simulink model "Controller_HIL"  (R2024a)
settings: Solver=FixedStepDiscrete  StartTime=0.0  StopTime=inf  FixedStep=ts_controller  RelTol=1e-3
InitFcn:
  | mbd_s32k_consistency_checks(bdroot(gcs));
undefined symbols (not defined in the file): Battery, BMS_Controller_State, Charging_State, currentFactor, CV_Gain, DiscIntNeverNeededParam, I_cc, LQFP, MaxCellVoltThrsld, noCurrent, Ns_Module, NumModules, OverCellVoltageLimit, SOCInit, SRE, ts_controller, ts_system, UnderCellVoltageLimit, voltThreshold
libraries: mbd_s32k1xx_ec_toolbox x104, etargetslib x95, mbd_bcc_ec_toolbox x30, hdlsllib x11, simulink x6, sharedTrackingLibrary x2
(part 2 of 4)

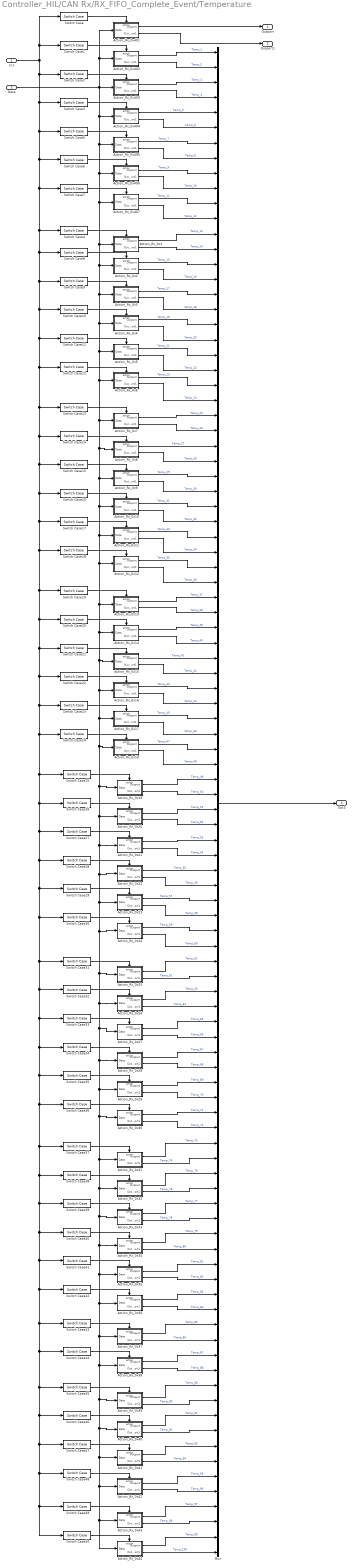
== system Controller_HIL/CAN Rx/RX_FIFO_Complete_Event/Temperature ==
  In1 : Inport
  Data : Inport  Port=2
  Action_Rx_0x1 : Subsystem  TreatAsAtomicUnit=on
  Action_Rx_0x10 : Subsystem  TreatAsAtomicUnit=on
  Action_Rx_0x11 : Subsystem  TreatAsAtomicUnit=on
  Action_Rx_0x12 : Subsystem  TreatAsAtomicUnit=on
  Action_Rx_0x13 : Subsystem  TreatAsAtomicUnit=on
  Action_Rx_0x14 : Subsystem  TreatAsAtomicUnit=on
  Action_Rx_0x15 : Subsystem  TreatAsAtomicUnit=on
  Action_Rx_0x16 : Subsystem  TreatAsAtomicUnit=on
  Action_Rx_0x17 : Subsystem  TreatAsAtomicUnit=on
  Action_Rx_0x18 : Subsystem  TreatAsAtomicUnit=on
  Action_Rx_0x19 : Subsystem  TreatAsAtomicUnit=on
  Action_Rx_0x2 : Subsystem  TreatAsAtomicUnit=on
  Action_Rx_0x20 : Subsystem  TreatAsAtomicUnit=on
  Action_Rx_0x21 : Subsystem  TreatAsAtomicUnit=on
  Action_Rx_0x22 : Subsystem  TreatAsAtomicUnit=on
  Action_Rx_0x23 : Subsystem  TreatAsAtomicUnit=on
  Action_Rx_0x24 : Subsystem  TreatAsAtomicUnit=on
  Action_Rx_0x25 : Subsystem  TreatAsAtomicUnit=on
  Action_Rx_0x26 : Subsystem  TreatAsAtomicUnit=on
  Action_Rx_0x27 : Subsystem  TreatAsAtomicUnit=on
  Action_Rx_0x28 : Subsystem  TreatAsAtomicUnit=on
  Action_Rx_0x29 : Subsystem  TreatAsAtomicUnit=on
  Action_Rx_0x3 : Subsystem  TreatAsAtomicUnit=on
  Action_Rx_0x30 : Subsystem  TreatAsAtomicUnit=on
  Action_Rx_0x31 : Subsystem  TreatAsAtomicUnit=on
  Action_Rx_0x32 : Subsystem  TreatAsAtomicUnit=on
  Action_Rx_0x33 : Subsystem  TreatAsAtomicUnit=on
  Action_Rx_0x34 : Subsystem  TreatAsAtomicUnit=on
  Action_Rx_0x35 : Subsystem  TreatAsAtomicUnit=on
  Action_Rx_0x36 : Subsystem  TreatAsAtomicUnit=on
  Action_Rx_0x37 : Subsystem  TreatAsAtomicUnit=on
  Action_Rx_0x38 : Subsystem  TreatAsAtomicUnit=on
  Action_Rx_0x39 : Subsystem  TreatAsAtomicUnit=on
  Action_Rx_0x4 : Subsystem  TreatAsAtomicUnit=on
  Action_Rx_0x40 : Subsystem  TreatAsAtomicUnit=on
  Action_Rx_0x401 : Subsystem  TreatAsAtomicUnit=on
  Action_Rx_0x402 : Subsystem  TreatAsAtomicUnit=on
  Action_Rx_0x403 : Subsystem  TreatAsAtomicUnit=on
  Action_Rx_0x404 : Subsystem  TreatAsAtomicUnit=on
  Action_Rx_0x405 : Subsystem  TreatAsAtomicUnit=on
  Action_Rx_0x406 : Subsystem  TreatAsAtomicUnit=on
  Action_Rx_0x407 : Subsystem  TreatAsAtomicUnit=on
  Action_Rx_0x41 : Subsystem  TreatAsAtomicUnit=on
  Action_Rx_0x42 : Subsystem  TreatAsAtomicUnit=on
  Action_Rx_0x43 : Subsystem  TreatAsAtomicUnit=on
  Action_Rx_0x44 : Subsystem  TreatAsAtomicUnit=on
  Action_Rx_0x5 : Subsystem  TreatAsAtomicUnit=on
  Action_Rx_0x6 : Subsystem  TreatAsAtomicUnit=on
  Action_Rx_0x7 : Subsystem  TreatAsAtomicUnit=on
  Action_Rx_0x8 : Subsystem  TreatAsAtomicUnit=on
  Action_Rx_0x9 : Subsystem  TreatAsAtomicUnit=on
  Mux : Mux  Inputs=100
  Switch Case : SwitchCase  CaseConditions={hex2dec('401')}  ShowDefaultCase=off
  Switch Case1 : SwitchCase  CaseConditions={hex2dec('402')}  ShowDefaultCase=off
  Switch Case10 : SwitchCase  CaseConditions={hex2dec('411')}  ShowDefaultCase=off
  Switch Case11 : SwitchCase  CaseConditions={hex2dec('412')}  ShowDefaultCase=off
  Switch Case12 : SwitchCase  CaseConditions={hex2dec('413')}  ShowDefaultCase=off
  Switch Case13 : SwitchCase  CaseConditions={hex2dec('414')}  ShowDefaultCase=off
  Switch Case14 : SwitchCase  CaseConditions={hex2dec('415')}  ShowDefaultCase=off
  Switch Case15 : SwitchCase  CaseConditions={hex2dec('416')}  ShowDefaultCase=off
  Switch Case16 : SwitchCase  CaseConditions={hex2dec('417')}  ShowDefaultCase=off
  Switch Case17 : SwitchCase  CaseConditions={hex2dec('418')}  ShowDefaultCase=off
  Switch Case18 : SwitchCase  CaseConditions={hex2dec('419')}  ShowDefaultCase=off
  Switch Case19 : SwitchCase  CaseConditions={hex2dec('420')}  ShowDefaultCase=off
  Switch Case2 : SwitchCase  CaseConditions={hex2dec('403')}  ShowDefaultCase=off
  Switch Case20 : SwitchCase  CaseConditions={hex2dec('421')}  ShowDefaultCase=off
  Switch Case21 : SwitchCase  CaseConditions={hex2dec('422')}  ShowDefaultCase=off
  Switch Case22 : SwitchCase  CaseConditions={hex2dec('423')}  ShowDefaultCase=off
  Switch Case23 : SwitchCase  CaseConditions={hex2dec('424')}  ShowDefaultCase=off
  Switch Case24 : SwitchCase  CaseConditions={hex2dec('425')}  ShowDefaultCase=off
  Switch Case25 : SwitchCase  CaseConditions={hex2dec('426')}  ShowDefaultCase=off
  Switch Case26 : SwitchCase  CaseConditions={hex2dec('427')}  ShowDefaultCase=off
  Switch Case27 : SwitchCase  CaseConditions={hex2dec('428')}  ShowDefaultCase=off
  Switch Case28 : SwitchCase  CaseConditions={hex2dec('429')}  ShowDefaultCase=off
  Switch Case29 : SwitchCase  CaseConditions={hex2dec('430')}  ShowDefaultCase=off
  Switch Case3 : SwitchCase  CaseConditions={hex2dec('404')}  ShowDefaultCase=off
  Switch Case30 : SwitchCase  CaseConditions={hex2dec('431')}  ShowDefaultCase=off
  Switch Case31 : SwitchCase  CaseConditions={hex2dec('432')}  ShowDefaultCase=off
  Switch Case32 : SwitchCase  CaseConditions={hex2dec('433')}  ShowDefaultCase=off
  Switch Case33 : SwitchCase  CaseConditions={hex2dec('434')}  ShowDefaultCase=off
  Switch Case34 : SwitchCase  CaseConditions={hex2dec('435')}  ShowDefaultCase=off
  Switch Case35 : SwitchCase  CaseConditions={hex2dec('436')}  ShowDefaultCase=off
  Switch Case36 : SwitchCase  CaseConditions={hex2dec('437')}  ShowDefaultCase=off
  Switch Case37 : SwitchCase  CaseConditions={hex2dec('438')}  ShowDefaultCase=off
  Switch Case38 : SwitchCase  CaseConditions={hex2dec('439')}  ShowDefaultCase=off
  Switch Case39 : SwitchCase  CaseConditions={hex2dec('440')}  ShowDefaultCase=off
  Switch Case4 : SwitchCase  CaseConditions={hex2dec('408')}  ShowDefaultCase=off
  Switch Case40 : SwitchCase  CaseConditions={hex2dec('441')}  ShowDefaultCase=off
  Switch Case41 : SwitchCase  CaseConditions={hex2dec('442')}  ShowDefaultCase=off
  Switch Case42 : SwitchCase  CaseConditions={hex2dec('443')}  ShowDefaultCase=off
  Switch Case43 : SwitchCase  CaseConditions={hex2dec('444')}  ShowDefaultCase=off
  Switch Case44 : SwitchCase  CaseConditions={hex2dec('445')}  ShowDefaultCase=off
  Switch Case45 : SwitchCase  CaseConditions={hex2dec('446')}  ShowDefaultCase=off
  Switch Case46 : SwitchCase  CaseConditions={hex2dec('447')}  ShowDefaultCase=off
  Switch Case47 : SwitchCase  CaseConditions={hex2dec('448')}  ShowDefaultCase=off
  Switch Case48 : SwitchCase  CaseConditions={hex2dec('449')}  ShowDefaultCase=off
  Switch Case49 : SwitchCase  CaseConditions={hex2dec('450')}  ShowDefaultCase=off
  Switch Case5 : SwitchCase  CaseConditions={hex2dec('405')}  ShowDefaultCase=off
  Switch Case50 : SwitchCase  CaseConditions={hex2dec('451')}  ShowDefaultCase=off
  Switch Case6 : SwitchCase  CaseConditions={hex2dec('406')}  ShowDefaultCase=off
  Switch Case7 : SwitchCase  CaseConditions={hex2dec('407')}  ShowDefaultCase=off
  Switch Case8 : SwitchCase  CaseConditions={hex2dec('409')}  ShowDefaultCase=off
  Switch Case9 : SwitchCase  CaseConditions={hex2dec('410')}  ShowDefaultCase=off
  Outport : Outport
  Outport1 : Outport  Port=2
  Out3 : Outport  Port=3
  wires:
  Action_Rx_0x35/1(Outport) -> Mux/81  "Temp_81"
  Action_Rx_0x19/2(Outport1) -> Mux/50  "Temp_50"
  Switch Case38/1 -> Action_Rx_0x32/Action
  In1/1 -> Switch Case3/1, Switch Case5/1, Switch Case6/1, Switch Case8/1, Switch Case9/1, Switch Case10/1, Switch Case11/1, Switch Case12/1, Switch Case13/1, Switch Case14/1, Switch Case15/1, Switch Case16/1, Switch Case18/1, Switch Case20/1, Switch Case21/1, Switch Case22/1, Switch Case23/1, Switch Case24/1, Switch Case25/1, Switch Case26/1, Switch Case28/1, Switch Case29/1, Switch Case31/1, Switch Case32/1, Switch Case33/1, Switch Case34/1, Switch Case35/1, Switch Case37/1, Switch Case38/1, Switch Case39/1, Switch Case40/1, Switch Case41/1, Switch Case45/1, Switch Case46/1, Switch Case48/1, Switch Case49/1, Switch Case50/1, Switch Case47/1, Switch Case44/1, Switch Case43/1, Switch Case42/1, Switch Case36/1, Switch Case30/1, Switch Case27/1, Switch Case19/1, Switch Case17/1, Switch Case4/1, Switch Case7/1, Switch Case2/1, Switch Case1/1, Switch Case/1
  Switch Case1/1 -> Action_Rx_0x402/Action
  Switch Case6/1 -> Action_Rx_0x406/Action
  Action_Rx_0x14/1(Outport) -> Mux/39  "Temp_39"
  Data/1 -> Action_Rx_0x405/1(Data), Action_Rx_0x406/1(Data), Action_Rx_0x3/1(Data), Action_Rx_0x4/1(Data), Action_Rx_0x5/1(Data), Action_Rx_0x7/1(Data), Action_Rx_0x8/1(Data), Action_Rx_0x9/1(Data), Action_Rx_0x10/1(Data), Action_Rx_0x11/1(Data), Action_Rx_0x12/1(Data), Action_Rx_0x13/1(Data), Action_Rx_0x14/1(Data), Action_Rx_0x15/1(Data), Action_Rx_0x16/1(Data), Action_Rx_0x17/1(Data), Action_Rx_0x18/1(Data), Action_Rx_0x19/1(Data), Action_Rx_0x20/1(Data), Action_Rx_0x21/1(Data), Action_Rx_0x22/1(Data), Action_Rx_0x23/1(Data), Action_Rx_0x24/1(Data), Action_Rx_0x25/1(Data), Action_Rx_0x26/1(Data), Action_Rx_0x27/1(Data), Action_Rx_0x28/1(Data), Action_Rx_0x29/1(Data), Action_Rx_0x30/1(Data), Action_Rx_0x31/1(Data), Action_Rx_0x32/1(Data), Action_Rx_0x33/1(Data), Action_Rx_0x34/1(Data), Action_Rx_0x35/1(Data), Action_Rx_0x36/1(Data), Action_Rx_0x37/1(Data), Action_Rx_0x39/1(Data), Action_Rx_0x40/1(Data), Action_Rx_0x41/1(Data), Action_Rx_0x42/1(Data), Action_Rx_0x43/1(Data), Action_Rx_0x44/1(Data), Action_Rx_0x38/1(Data), Action_Rx_0x6/1(Data), Action_Rx_0x2/1(Data), Action_Rx_0x1/1(Data), Action_Rx_0x407/1(Data), Action_Rx_0x404/1(Data), Action_Rx_0x403/1(Data), Action_Rx_0x402/1(Data), Action_Rx_0x401/1(Data)
  Switch Case43/1 -> Action_Rx_0x37/Action
  Action_Rx_0x13/1(Outport) -> Mux/37  "Temp_37"
  Switch Case2/1 -> Action_Rx_0x403/Action
  Action_Rx_0x34/1(Outport) -> Mux/79  "Temp_79"
  Action_Rx_0x5/1(Outport) -> Mux/21  "Temp_21"
  Action_Rx_0x44/2(Outport1) -> Mux/100  "Temp_100"
  Action_Rx_0x15/1(Outport) -> Mux/41  "Temp_41"
  Switch Case18/1 -> Action_Rx_0x12/Action
  Action_Rx_0x31/1(Outport) -> Mux/73  "Temp_73"
  Switch Case7/1 -> Action_Rx_0x407/Action
  Switch Case47/1 -> Action_Rx_0x41/Action
  Switch Case14/1 -> Action_Rx_0x8/Action
  Action_Rx_0x405/1(Outport) -> Mux/7  "Temp_7"
  Switch Case20/1 -> Action_Rx_0x14/Action
  Action_Rx_0x4/1(Outport) -> Mux/19  "Temp_19"
  Action_Rx_0x402/2(Outport1) -> Mux/2  "Temp_2"
  Switch Case3/1 -> Action_Rx_0x404/Action
  Action_Rx_0x20/1(Outport) -> Mux/51  "Temp_51"
  Action_Rx_0x17/2(Outport1) -> Mux/46  "Temp_46"
  Switch Case8/1 -> Action_Rx_0x2/Action
  Action_Rx_0x21/1(Outport) -> Mux/53  "Temp_53"
  Switch Case50/1 -> Action_Rx_0x44/Action
  Action_Rx_0x43/2(Outport1) -> Mux/98  "Temp_98"
  Mux/1 -> Out3/1
  Action_Rx_0x40/2(Outport1) -> Mux/92  "Temp_92"
  Switch Case13/1 -> Action_Rx_0x7/Action
  Action_Rx_0x32/1(Outport) -> Mux/75  "Temp_75"
  Switch Case21/1 -> Action_Rx_0x15/Action
  Switch Case35/1 -> Action_Rx_0x29/Action
  Action_Rx_0x406/2(Outport1) -> Mux/10  "Temp_10"
  Action_Rx_0x25/1(Outport) -> Mux/61  "Temp_61"
  Switch Case32/1 -> Action_Rx_0x26/Action
  Action_Rx_0x403/1(Outport) -> Mux/3  "Temp_3"
  Action_Rx_0x6/1(Outport) -> Mux/23  "Temp_23"
  Action_Rx_0x36/2(Outport1) -> Mux/84  "Temp_84"
  Action_Rx_0x1/2(Outport1) -> Mux/14  "Temp_14"
  Action_Rx_0x18/2(Outport1) -> Mux/48  "Temp_48"
  Action_Rx_0x404/2(Outport1) -> Mux/6  "Temp_6"
  Action_Rx_0x2/2(Outport1) -> Mux/16  "Temp_16"
  Action_Rx_0x405/2(Outport1) -> Mux/8  "Temp_8"
  Action_Rx_0x42/2(Outport1) -> Mux/96  "Temp_96"
  Action_Rx_0x9/2(Outport1) -> Mux/30  "Temp_30"
  Action_Rx_0x13/2(Outport1) -> Mux/38  "Temp_38"
  Action_Rx_0x15/2(Outport1) -> Mux/42  "Temp_42"
  Switch Case16/1 -> Action_Rx_0x10/Action
  Action_Rx_0x34/2(Outport1) -> Mux/80  "Temp_80"
  Switch Case9/1 -> Action_Rx_0x3/Action
  Switch Case27/1 -> Action_Rx_0x21/Action
  Switch Case30/1 -> Action_Rx_0x24/Action
  Action_Rx_0x4/2(Outport1) -> Mux/20  "Temp_20"
  Action_Rx_0x16/2(Outport1) -> Mux/44  "Temp_44"
  Switch Case31/1 -> Action_Rx_0x25/Action
  Action_Rx_0x407/1(Outport) -> Mux/11  "Temp_11"
  Switch Case45/1 -> Action_Rx_0x39/Action
  Switch Case33/1 -> Action_Rx_0x27/Action
  Action_Rx_0x38/1(Outport) -> Mux/87  "Temp_87"
  Switch Case22/1 -> Action_Rx_0x16/Action
  Switch Case12/1 -> Action_Rx_0x6/Action
  Switch Case41/1 -> Action_Rx_0x35/Action
  Switch Case19/1 -> Action_Rx_0x13/Action
  Action_Rx_0x403/2(Outport1) -> Mux/4  "Temp_4"
  Switch Case29/1 -> Action_Rx_0x23/Action
  Action_Rx_0x22/1(Outport) -> Mux/55  "Temp_55"
  Switch Case39/1 -> Action_Rx_0x33/Action
  Action_Rx_0x407/2(Outport1) -> Mux/12  "Temp_12"
  Switch Case/1 -> Action_Rx_0x401/Action
  Action_Rx_0x20/2(Outport1) -> Mux/52  "Temp_52"
  Action_Rx_0x16/1(Outport) -> Mux/43  "Temp_43"
  Action_Rx_0x10/1(Outport) -> Mux/31  "Temp_31"
  Switch Case4/1 -> Action_Rx_0x1/Action
  Action_Rx_0x28/1(Outport) -> Mux/67  "Temp_67"
  Switch Case17/1 -> Action_Rx_0x11/Action
  Switch Case46/1 -> Action_Rx_0x40/Action
  Action_Rx_0x22/2(Outport1) -> Mux/56  "Temp_56"
  Action_Rx_0x26/1(Outport) -> Mux/63  "Temp_63"
  Action_Rx_0x7/2(Outport1) -> Mux/26  "Temp_26"
  Action_Rx_0x26/2(Outport1) -> Mux/64  "Temp_64"
  Action_Rx_0x3/2(Outport1) -> Mux/18  "Temp_18"
  Action_Rx_0x38/2(Outport1) -> Mux/88  "Temp_88"
  Switch Case49/1 -> Action_Rx_0x43/Action
  Action_Rx_0x41/2(Outport1) -> Mux/94  "Temp_94"
  Action_Rx_0x23/1(Outport) -> Mux/57  "Temp_57"
  Action_Rx_0x25/2(Outport1) -> Mux/62  "Temp_62"
  Action_Rx_0x37/1(Outport) -> Mux/85  "Temp_85"
  Action_Rx_0x27/2(Outport1) -> Mux/66  "Temp_66"
  Action_Rx_0x35/2(Outport1) -> Mux/82  "Temp_82"
  Action_Rx_0x33/1(Outport) -> Mux/77  "Temp_77"
  Action_Rx_0x29/1(Outport) -> Mux/69  "Temp_69"
  Action_Rx_0x8/1(Outport) -> Mux/27  "Temp_27"
  Action_Rx_0x404/1(Outport) -> Mux/5  "Temp_5"
  Action_Rx_0x30/1(Outport) -> Mux/71  "Temp_71"
  Switch Case5/1 -> Action_Rx_0x405/Action
  Switch Case26/1 -> Action_Rx_0x20/Action
  Action_Rx_0x28/2(Outport1) -> Mux/68  "Temp_68"
  Switch Case48/1 -> Action_Rx_0x42/Action
  Action_Rx_0x39/2(Outport1) -> Mux/90  "Temp_90"
  Action_Rx_0x406/1(Outport) -> Mux/9  "Temp_9"
  Action_Rx_0x9/1(Outport) -> Mux/29  "Temp_29"
  Action_Rx_0x7/1(Outport) -> Mux/25  "Temp_25"
  Action_Rx_0x24/1(Outport) -> Mux/59  "Temp_59"
  Switch Case25/1 -> Action_Rx_0x19/Action
  Action_Rx_0x32/2(Outport1) -> Mux/76  "Temp_76"
  Action_Rx_0x1/1(Outport) -> Mux/13  "Temp_13"
  Action_Rx_0x29/2(Outport1) -> Mux/70  "Temp_70"
  Action_Rx_0x31/2(Outport1) -> Mux/74  "Temp_74"
  Switch Case42/1 -> Action_Rx_0x36/Action
  Switch Case23/1 -> Action_Rx_0x17/Action
  Action_Rx_0x33/2(Outport1) -> Mux/78  "Temp_78"
  Action_Rx_0x36/1(Outport) -> Mux/83  "Temp_83"
  Switch Case37/1 -> Action_Rx_0x31/Action
  Switch Case44/1 -> Action_Rx_0x38/Action
  Switch Case24/1 -> Action_Rx_0x18/Action
  Action_Rx_0x21/2(Outport1) -> Mux/54  "Temp_54"
  Action_Rx_0x11/1(Outport) -> Mux/33  "Temp_33"
  Action_Rx_0x401/2(Outport1) -> Outport1/1
  Action_Rx_0x41/1(Outport) -> Mux/93  "Temp_93"
  Switch Case34/1 -> Action_Rx_0x28/Action
  Switch Case36/1 -> Action_Rx_0x30/Action
  Action_Rx_0x37/2(Outport1) -> Mux/86  "Temp_86"
  Action_Rx_0x27/1(Outport) -> Mux/65  "Temp_65"
  Action_Rx_0x44/1(Outport) -> Mux/99  "Temp_99"
  Action_Rx_0x14/2(Outport1) -> Mux/40  "Temp_40"
  Action_Rx_0x40/1(Outport) -> Mux/91  "Temp_91"
  Action_Rx_0x402/1(Outport) -> Mux/1  "Temp_1"
  Switch Case15/1 -> Action_Rx_0x9/Action
  Action_Rx_0x12/1(Outport) -> Mux/35  "Temp_35"
  Switch Case28/1 -> Action_Rx_0x22/Action
  Switch Case40/1 -> Action_Rx_0x34/Action
  Action_Rx_0x24/2(Outport1) -> Mux/60  "Temp_60"
  Action_Rx_0x23/2(Outport1) -> Mux/58  "Temp_58"
  Action_Rx_0x17/1(Outport) -> Mux/45  "Temp_45"
  Action_Rx_0x18/1(Outport) -> Mux/47  "Temp_47"
  Action_Rx_0x8/2(Outport1) -> Mux/28  "Temp_28"
  Action_Rx_0x6/2(Outport1) -> Mux/24  "Temp_24"
  Action_Rx_0x39/1(Outport) -> Mux/89  "Temp_89"
  Action_Rx_0x5/2(Outport1) -> Mux/22  "Temp_22"
  Action_Rx_0x43/1(Outport) -> Mux/97  "Temp_97"
  Action_Rx_0x42/1(Outport) -> Mux/95  "Temp_95"
  Action_Rx_0x19/1(Outport) -> Mux/49  "Temp_49"
  Action_Rx_0x30/2(Outport1) -> Mux/72  "Temp_72"
  Switch Case11/1 -> Action_Rx_0x5/Action
  Action_Rx_0x2/1(Outport) -> Mux/15  "Temp_15"
  Action_Rx_0x3/1(Outport) -> Mux/17  "Temp_17"
  Action_Rx_0x11/2(Outport1) -> Mux/34  "Temp_34"
  Switch Case10/1 -> Action_Rx_0x4/Action
  Action_Rx_0x12/2(Outport1) -> Mux/36  "Temp_36"
  Action_Rx_0x10/2(Outport1) -> Mux/32  "Temp_32"
  Action_Rx_0x401/1(Outport) -> Outport/1

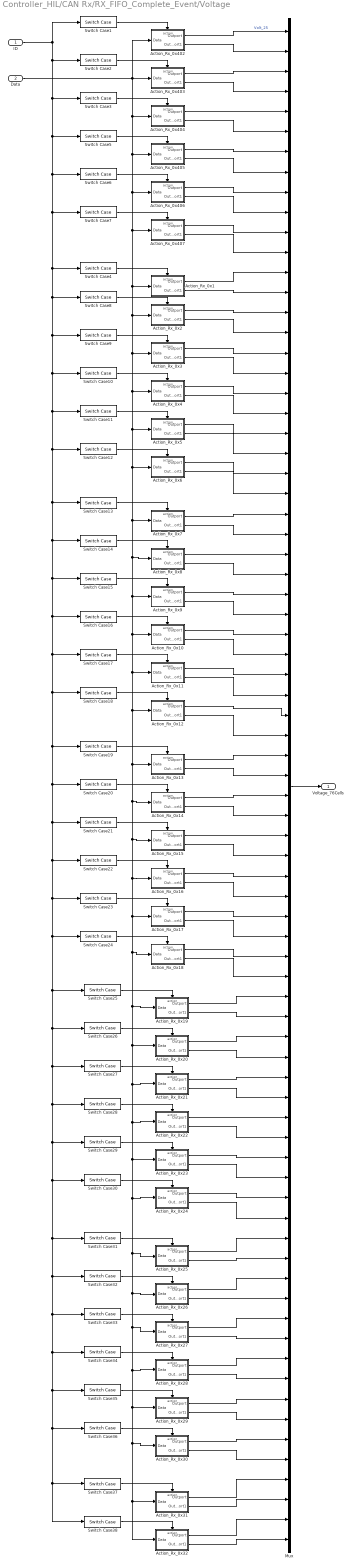
== system Controller_HIL/CAN Rx/RX_FIFO_Complete_Event/Voltage ==
  ID : Inport
  Data : Inport  Port=2
  Action_Rx_0x1 : Subsystem  TreatAsAtomicUnit=on
  Action_Rx_0x10 : Subsystem  TreatAsAtomicUnit=on
  Action_Rx_0x11 : Subsystem  TreatAsAtomicUnit=on
  Action_Rx_0x12 : Subsystem  TreatAsAtomicUnit=on
  Action_Rx_0x13 : Subsystem  TreatAsAtomicUnit=on
  Action_Rx_0x14 : Subsystem  TreatAsAtomicUnit=on
  Action_Rx_0x15 : Subsystem  TreatAsAtomicUnit=on
  Action_Rx_0x16 : Subsystem  TreatAsAtomicUnit=on
  Action_Rx_0x17 : Subsystem  TreatAsAtomicUnit=on
  Action_Rx_0x18 : Subsystem  TreatAsAtomicUnit=on
  Action_Rx_0x19 : Subsystem  TreatAsAtomicUnit=on
  Action_Rx_0x2 : Subsystem  TreatAsAtomicUnit=on
  Action_Rx_0x20 : Subsystem  TreatAsAtomicUnit=on
  Action_Rx_0x21 : Subsystem  TreatAsAtomicUnit=on
  Action_Rx_0x22 : Subsystem  TreatAsAtomicUnit=on
  Action_Rx_0x23 : Subsystem  TreatAsAtomicUnit=on
  Action_Rx_0x24 : Subsystem  TreatAsAtomicUnit=on
  Action_Rx_0x25 : Subsystem  TreatAsAtomicUnit=on
  Action_Rx_0x26 : Subsystem  TreatAsAtomicUnit=on
  Action_Rx_0x27 : Subsystem  TreatAsAtomicUnit=on
  Action_Rx_0x28 : Subsystem  TreatAsAtomicUnit=on
  Action_Rx_0x29 : Subsystem  TreatAsAtomicUnit=on
  Action_Rx_0x3 : Subsystem  TreatAsAtomicUnit=on
  Action_Rx_0x30 : Subsystem  TreatAsAtomicUnit=on
  Action_Rx_0x31 : Subsystem  TreatAsAtomicUnit=on
  Action_Rx_0x32 : Subsystem  TreatAsAtomicUnit=on
  Action_Rx_0x4 : Subsystem  TreatAsAtomicUnit=on
  Action_Rx_0x402 : Subsystem  TreatAsAtomicUnit=on
  Action_Rx_0x403 : Subsystem  TreatAsAtomicUnit=on
  Action_Rx_0x404 : Subsystem  TreatAsAtomicUnit=on
  Action_Rx_0x405 : Subsystem  TreatAsAtomicUnit=on
  Action_Rx_0x406 : Subsystem  TreatAsAtomicUnit=on
  Action_Rx_0x407 : Subsystem  TreatAsAtomicUnit=on
  Action_Rx_0x5 : Subsystem  TreatAsAtomicUnit=on
  Action_Rx_0x6 : Subsystem  TreatAsAtomicUnit=on
  Action_Rx_0x7 : Subsystem  TreatAsAtomicUnit=on
  Action_Rx_0x8 : Subsystem  TreatAsAtomicUnit=on
  Action_Rx_0x9 : Subsystem  TreatAsAtomicUnit=on
  Mux : Mux  Inputs=76
  Switch Case1 : SwitchCase  CaseConditions={hex2dec('452')}  ShowDefaultCase=off
  Switch Case10 : SwitchCase  CaseConditions={hex2dec('461')}  ShowDefaultCase=off
  Switch Case11 : SwitchCase  CaseConditions={hex2dec('462')}  ShowDefaultCase=off
  Switch Case12 : SwitchCase  CaseConditions={hex2dec('463')}  ShowDefaultCase=off
  Switch Case13 : SwitchCase  CaseConditions={hex2dec('464')}  ShowDefaultCase=off
  Switch Case14 : SwitchCase  CaseConditions={hex2dec('465')}  ShowDefaultCase=off
  Switch Case15 : SwitchCase  CaseConditions={hex2dec('466')}  ShowDefaultCase=off
  Switch Case16 : SwitchCase  CaseConditions={hex2dec('467')}  ShowDefaultCase=off
  Switch Case17 : SwitchCase  CaseConditions={hex2dec('468')}  ShowDefaultCase=off
  Switch Case18 : SwitchCase  CaseConditions={hex2dec('469')}  ShowDefaultCase=off
  Switch Case19 : SwitchCase  CaseConditions={hex2dec('470')}  ShowDefaultCase=off
  Switch Case2 : SwitchCase  CaseConditions={hex2dec('453')}  ShowDefaultCase=off
  Switch Case20 : SwitchCase  CaseConditions={hex2dec('471')}  ShowDefaultCase=off
  Switch Case21 : SwitchCase  CaseConditions={hex2dec('472')}  ShowDefaultCase=off
  Switch Case22 : SwitchCase  CaseConditions={hex2dec('473')}  ShowDefaultCase=off
  Switch Case23 : SwitchCase  CaseConditions={hex2dec('474')}  ShowDefaultCase=off
  Switch Case24 : SwitchCase  CaseConditions={hex2dec('475')}  ShowDefaultCase=off
  Switch Case25 : SwitchCase  CaseConditions={hex2dec('476')}  ShowDefaultCase=off
  Switch Case26 : SwitchCase  CaseConditions={hex2dec('477')}  ShowDefaultCase=off
  Switch Case27 : SwitchCase  CaseConditions={hex2dec('478')}  ShowDefaultCase=off
  Switch Case28 : SwitchCase  CaseConditions={hex2dec('479')}  ShowDefaultCase=off
  Switch Case29 : SwitchCase  CaseConditions={hex2dec('480')}  ShowDefaultCase=off
  Switch Case3 : SwitchCase  CaseConditions={hex2dec('454')}  ShowDefaultCase=off
  Switch Case30 : SwitchCase  CaseConditions={hex2dec('481')}  ShowDefaultCase=off
  Switch Case31 : SwitchCase  CaseConditions={hex2dec('482')}  ShowDefaultCase=off
  Switch Case32 : SwitchCase  CaseConditions={hex2dec('483')}  ShowDefaultCase=off
  Switch Case33 : SwitchCase  CaseConditions={hex2dec('484')}  ShowDefaultCase=off
  Switch Case34 : SwitchCase  CaseConditions={hex2dec('485')}  ShowDefaultCase=off
  Switch Case35 : SwitchCase  CaseConditions={hex2dec('486')}  ShowDefaultCase=off
  Switch Case36 : SwitchCase  CaseConditions={hex2dec('487')}  ShowDefaultCase=off
  Switch Case37 : SwitchCase  CaseConditions={hex2dec('488')}  ShowDefaultCase=off
  Switch Case38 : SwitchCase  CaseConditions={hex2dec('489')}  ShowDefaultCase=off
  Switch Case4 : SwitchCase  CaseConditions={hex2dec('458')}  ShowDefaultCase=off
  Switch Case5 : SwitchCase  CaseConditions={hex2dec('455')}  ShowDefaultCase=off
  Switch Case6 : SwitchCase  CaseConditions={hex2dec('456')}  ShowDefaultCase=off
  Switch Case7 : SwitchCase  CaseConditions={hex2dec('457')}  ShowDefaultCase=off
  Switch Case8 : SwitchCase  CaseConditions={hex2dec('459')}  ShowDefaultCase=off
  Switch Case9 : SwitchCase  CaseConditions={hex2dec('460')}  ShowDefaultCase=off
  Voltage_76Cells : Outport
  wires:
  Action_Rx_0x19/2(Outport1) -> Mux/50
  Switch Case38/1 -> Action_Rx_0x32/Action
  ID/1 -> Switch Case3/1, Switch Case5/1, Switch Case6/1, Switch Case8/1, Switch Case9/1, Switch Case10/1, Switch Case11/1, Switch Case12/1, Switch Case13/1, Switch Case14/1, Switch Case15/1, Switch Case16/1, Switch Case18/1, Switch Case20/1, Switch Case21/1, Switch Case22/1, Switch Case23/1, Switch Case24/1, Switch Case25/1, Switch Case26/1, Switch Case28/1, Switch Case29/1, Switch Case31/1, Switch Case32/1, Switch Case33/1, Switch Case34/1, Switch Case35/1, Switch Case37/1, Switch Case38/1, Switch Case36/1, Switch Case30/1, Switch Case27/1, Switch Case19/1, Switch Case17/1, Switch Case4/1, Switch Case7/1, Switch Case2/1, Switch Case1/1
  Switch Case1/1 -> Action_Rx_0x402/Action
  Switch Case6/1 -> Action_Rx_0x406/Action
  Action_Rx_0x14/1(Outport) -> Mux/39
  Data/1 -> Action_Rx_0x405/1(Data), Action_Rx_0x406/1(Data), Action_Rx_0x3/1(Data), Action_Rx_0x4/1(Data), Action_Rx_0x5/1(Data), Action_Rx_0x7/1(Data), Action_Rx_0x8/1(Data), Action_Rx_0x9/1(Data), Action_Rx_0x10/1(Data), Action_Rx_0x11/1(Data), Action_Rx_0x12/1(Data), Action_Rx_0x13/1(Data), Action_Rx_0x14/1(Data), Action_Rx_0x15/1(Data), Action_Rx_0x16/1(Data), Action_Rx_0x17/1(Data), Action_Rx_0x18/1(Data), Action_Rx_0x19/1(Data), Action_Rx_0x20/1(Data), Action_Rx_0x21/1(Data), Action_Rx_0x22/1(Data), Action_Rx_0x23/1(Data), Action_Rx_0x24/1(Data), Action_Rx_0x25/1(Data), Action_Rx_0x26/1(Data), Action_Rx_0x27/1(Data), Action_Rx_0x28/1(Data), Action_Rx_0x29/1(Data), Action_Rx_0x30/1(Data), Action_Rx_0x31/1(Data), Action_Rx_0x32/1(Data), Action_Rx_0x6/1(Data), Action_Rx_0x2/1(Data), Action_Rx_0x1/1(Data), Action_Rx_0x407/1(Data), Action_Rx_0x404/1(Data), Action_Rx_0x403/1(Data), Action_Rx_0x402/1(Data)
  Action_Rx_0x13/1(Outport) -> Mux/37
  Switch Case2/1 -> Action_Rx_0x403/Action
  Action_Rx_0x5/1(Outport) -> Mux/21
  Action_Rx_0x15/1(Outport) -> Mux/41
  Switch Case18/1 -> Action_Rx_0x12/Action
  Action_Rx_0x31/1(Outport) -> Mux/73
  Switch Case7/1 -> Action_Rx_0x407/Action
  Switch Case14/1 -> Action_Rx_0x8/Action
  Action_Rx_0x405/1(Outport) -> Mux/7
  Switch Case20/1 -> Action_Rx_0x14/Action
  Action_Rx_0x4/1(Outport) -> Mux/19
  Action_Rx_0x402/2(Outport1) -> Mux/2
  Switch Case3/1 -> Action_Rx_0x404/Action
  Action_Rx_0x20/1(Outport) -> Mux/51
  Action_Rx_0x17/2(Outport1) -> Mux/46
  Switch Case8/1 -> Action_Rx_0x2/Action
  Action_Rx_0x21/1(Outport) -> Mux/53
  Mux/1 -> Voltage_76Cells/1
  Switch Case13/1 -> Action_Rx_0x7/Action
  Action_Rx_0x32/1(Outport) -> Mux/75
  Switch Case21/1 -> Action_Rx_0x15/Action
  Switch Case35/1 -> Action_Rx_0x29/Action
  Action_Rx_0x406/2(Outport1) -> Mux/10
  Action_Rx_0x25/1(Outport) -> Mux/61
  Switch Case32/1 -> Action_Rx_0x26/Action
  Action_Rx_0x403/1(Outport) -> Mux/3
  Action_Rx_0x6/1(Outport) -> Mux/23
  Action_Rx_0x1/2(Outport1) -> Mux/14
  Action_Rx_0x18/2(Outport1) -> Mux/48
  Action_Rx_0x404/2(Outport1) -> Mux/6
  Action_Rx_0x2/2(Outport1) -> Mux/16
  Action_Rx_0x405/2(Outport1) -> Mux/8
  Action_Rx_0x9/2(Outport1) -> Mux/30
  Action_Rx_0x13/2(Outport1) -> Mux/38
  Action_Rx_0x15/2(Outport1) -> Mux/42
  Switch Case16/1 -> Action_Rx_0x10/Action
  Switch Case9/1 -> Action_Rx_0x3/Action
  Switch Case27/1 -> Action_Rx_0x21/Action
  Switch Case30/1 -> Action_Rx_0x24/Action
  Action_Rx_0x4/2(Outport1) -> Mux/20
  Action_Rx_0x16/2(Outport1) -> Mux/44
  Switch Case31/1 -> Action_Rx_0x25/Action
  Action_Rx_0x407/1(Outport) -> Mux/11
  Switch Case33/1 -> Action_Rx_0x27/Action
  Switch Case22/1 -> Action_Rx_0x16/Action
  Switch Case12/1 -> Action_Rx_0x6/Action
  Switch Case19/1 -> Action_Rx_0x13/Action
  Action_Rx_0x403/2(Outport1) -> Mux/4
  Switch Case29/1 -> Action_Rx_0x23/Action
  Action_Rx_0x22/1(Outport) -> Mux/55
  Action_Rx_0x407/2(Outport1) -> Mux/12
  Action_Rx_0x20/2(Outport1) -> Mux/52
  Action_Rx_0x16/1(Outport) -> Mux/43
  Action_Rx_0x10/1(Outport) -> Mux/31
  Switch Case4/1 -> Action_Rx_0x1/Action
  Action_Rx_0x28/1(Outport) -> Mux/67
  Switch Case17/1 -> Action_Rx_0x11/Action
  Action_Rx_0x22/2(Outport1) -> Mux/56
  Action_Rx_0x26/1(Outport) -> Mux/63
  Action_Rx_0x7/2(Outport1) -> Mux/26
  Action_Rx_0x26/2(Outport1) -> Mux/64
  Action_Rx_0x3/2(Outport1) -> Mux/18
  Action_Rx_0x23/1(Outport) -> Mux/57
  Action_Rx_0x25/2(Outport1) -> Mux/62
  Action_Rx_0x27/2(Outport1) -> Mux/66
  Action_Rx_0x29/1(Outport) -> Mux/69
  Action_Rx_0x8/1(Outport) -> Mux/27
  Action_Rx_0x404/1(Outport) -> Mux/5
  Action_Rx_0x30/1(Outport) -> Mux/71
  Switch Case5/1 -> Action_Rx_0x405/Action
  Switch Case26/1 -> Action_Rx_0x20/Action
  Action_Rx_0x28/2(Outport1) -> Mux/68
  Action_Rx_0x406/1(Outport) -> Mux/9
  Action_Rx_0x9/1(Outport) -> Mux/29
  Action_Rx_0x7/1(Outport) -> Mux/25
  Action_Rx_0x24/1(Outport) -> Mux/59
  Switch Case25/1 -> Action_Rx_0x19/Action
  Action_Rx_0x32/2(Outport1) -> Mux/76
  Action_Rx_0x1/1(Outport) -> Mux/13
  Action_Rx_0x29/2(Outport1) -> Mux/70
  Action_Rx_0x31/2(Outport1) -> Mux/74
  Switch Case23/1 -> Action_Rx_0x17/Action
  Switch Case37/1 -> Action_Rx_0x31/Action
  Switch Case24/1 -> Action_Rx_0x18/Action
  Action_Rx_0x21/2(Outport1) -> Mux/54
  Action_Rx_0x11/1(Outport) -> Mux/33
  Switch Case34/1 -> Action_Rx_0x28/Action
  Switch Case36/1 -> Action_Rx_0x30/Action
  Action_Rx_0x27/1(Outport) -> Mux/65
  Action_Rx_0x14/2(Outport1) -> Mux/40
  Action_Rx_0x402/1(Outport) -> Mux/1  "Volt_25"
  Switch Case15/1 -> Action_Rx_0x9/Action
  Action_Rx_0x12/1(Outport) -> Mux/35
  Switch Case28/1 -> Action_Rx_0x22/Action
  Action_Rx_0x24/2(Outport1) -> Mux/60
  Action_Rx_0x23/2(Outport1) -> Mux/58
  Action_Rx_0x17/1(Outport) -> Mux/45
  Action_Rx_0x18/1(Outport) -> Mux/47
  Action_Rx_0x8/2(Outport1) -> Mux/28
  Action_Rx_0x6/2(Outport1) -> Mux/24
  Action_Rx_0x5/2(Outport1) -> Mux/22
  Action_Rx_0x19/1(Outport) -> Mux/49
  Action_Rx_0x30/2(Outport1) -> Mux/72
  Switch Case11/1 -> Action_Rx_0x5/Action
  Action_Rx_0x2/1(Outport) -> Mux/15
  Action_Rx_0x3/1(Outport) -> Mux/17
  Action_Rx_0x11/2(Outport1) -> Mux/34
  Switch Case10/1 -> Action_Rx_0x4/Action
  Action_Rx_0x12/2(Outport1) -> Mux/36
  Action_Rx_0x10/2(Outport1) -> Mux/32

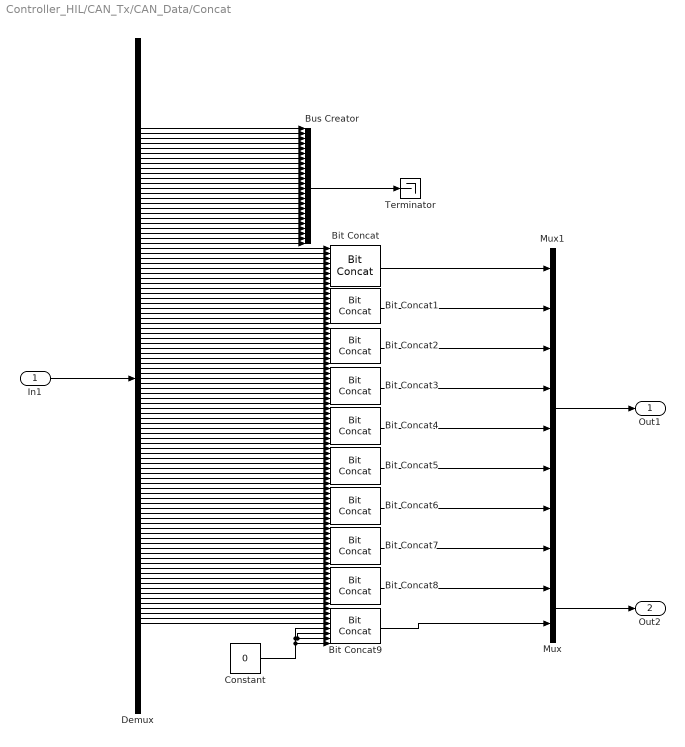
== system Controller_HIL/CAN_Tx/CAN_Data/Concat ==
  In1 : Inport
  Bit Concat{,1..9} (10 alike) : hdlsllib/Logic and Bit Operations/Bit Concat  numInputs=8
  Bus Creator : BusCreator  Inputs=24
  Constant : Constant  Value=0  OutDataTypeStr=boolean
  Demux : Demux  Outputs=100
  Mux : Mux  Inputs=2
  Mux1 : Mux  Inputs=8
  Terminator : Terminator
  Out1 : Outport
  Out2 : Outport  Port=2
  wires:
  In1/1 -> Demux/1
  Demux/1 -> Bus Creator/1
  Demux/2 -> Bus Creator/2
  Demux/3 -> Bus Creator/3
  Demux/4 -> Bus Creator/4
  Demux/5 -> Bus Creator/5
  Demux/6 -> Bus Creator/6
  Demux/7 -> Bus Creator/7
  Demux/8 -> Bus Creator/8
  Demux/9 -> Bus Creator/9
  Demux/10 -> Bus Creator/10
  Demux/11 -> Bus Creator/11
  Demux/12 -> Bus Creator/12
  Demux/13 -> Bus Creator/13
  Demux/14 -> Bus Creator/14
  Demux/15 -> Bus Creator/15
  Demux/16 -> Bus Creator/16
  Demux/17 -> Bus Creator/17
  Demux/18 -> Bus Creator/18
  Demux/19 -> Bus Creator/19
  Demux/20 -> Bus Creator/20
  Demux/21 -> Bus Creator/21
  Demux/22 -> Bus Creator/22
  Demux/23 -> Bus Creator/23
  Demux/24 -> Bus Creator/24
  Demux/25 -> Bit Concat/1
  Demux/26 -> Bit Concat/2
  Demux/27 -> Bit Concat/3
  Demux/28 -> Bit Concat/4
  Demux/29 -> Bit Concat/5
  Demux/30 -> Bit Concat/6
  Demux/31 -> Bit Concat/7
  Demux/32 -> Bit Concat/8
  Demux/33 -> Bit Concat1/1
  Demux/34 -> Bit Concat1/2
  Demux/35 -> Bit Concat1/3
  Demux/36 -> Bit Concat1/4
  Demux/37 -> Bit Concat1/5
  Demux/38 -> Bit Concat1/6
  Demux/39 -> Bit Concat1/7
  Demux/40 -> Bit Concat1/8
  Demux/41 -> Bit Concat2/1
  Demux/42 -> Bit Concat2/2
  Demux/43 -> Bit Concat2/3
  Demux/44 -> Bit Concat2/4
  Demux/45 -> Bit Concat2/5
  Demux/46 -> Bit Concat2/6
  Demux/47 -> Bit Concat2/7
  Demux/48 -> Bit Concat2/8
  Demux/49 -> Bit Concat3/1
  Demux/50 -> Bit Concat3/2
  Demux/51 -> Bit Concat3/3
  Demux/52 -> Bit Concat3/4
  Demux/53 -> Bit Concat3/5
  Demux/54 -> Bit Concat3/6
  Demux/55 -> Bit Concat3/7
  Demux/56 -> Bit Concat3/8
  Demux/57 -> Bit Concat4/1
  Demux/58 -> Bit Concat4/2
  Demux/59 -> Bit Concat4/3
  Demux/60 -> Bit Concat4/4
  Demux/61 -> Bit Concat4/5
  Demux/62 -> Bit Concat4/6
  Demux/63 -> Bit Concat4/7
  Demux/64 -> Bit Concat4/8
  Demux/65 -> Bit Concat5/1
  Demux/66 -> Bit Concat5/2
  Demux/67 -> Bit Concat5/3
  Demux/68 -> Bit Concat5/4
  Demux/69 -> Bit Concat5/5
  Demux/70 -> Bit Concat5/6
  Demux/71 -> Bit Concat5/7
  Demux/72 -> Bit Concat5/8
  Demux/73 -> Bit Concat6/1
  Demux/74 -> Bit Concat6/2
  Demux/75 -> Bit Concat6/3
  Demux/76 -> Bit Concat6/4
  Demux/77 -> Bit Concat6/5
  Demux/78 -> Bit Concat6/6
  Demux/79 -> Bit Concat6/7
  Demux/80 -> Bit Concat6/8
  Demux/81 -> Bit Concat7/1
  Demux/82 -> Bit Concat7/2
  Demux/83 -> Bit Concat7/3
  Demux/84 -> Bit Concat7/4
  Demux/85 -> Bit Concat7/5
  Demux/86 -> Bit Concat7/6
  Demux/87 -> Bit Concat7/7
  Demux/88 -> Bit Concat7/8
  Demux/89 -> Bit Concat8/1
  Demux/90 -> Bit Concat8/2
  Demux/91 -> Bit Concat8/3
  Demux/92 -> Bit Concat8/4
  Demux/93 -> Bit Concat8/5
  Demux/94 -> Bit Concat8/6
  Demux/95 -> Bit Concat8/7
  Demux/96 -> Bit Concat8/8
  Bus Creator/1 -> Terminator/1
  Demux/97 -> Bit Concat9/1
  Demux/98 -> Bit Concat9/2
  Demux/99 -> Bit Concat9/3
  Demux/100 -> Bit Concat9/4
  Constant/1 -> Bit Concat9/8, Bit Concat9/5, Bit Concat9/6, Bit Concat9/7
  Bit Concat/1 -> Mux1/1
  Bit Concat1/1 -> Mux1/2
  Bit Concat2/1 -> Mux1/3
  Bit Concat3/1 -> Mux1/4
  Bit Concat4/1 -> Mux1/5
  Bit Concat5/1 -> Mux1/6
  Bit Concat6/1 -> Mux1/7
  Bit Concat7/1 -> Mux1/8
  Mux1/1 -> Out1/1
  Bit Concat8/1 -> Mux/1
  Bit Concat9/1 -> Mux/2
  Mux/1 -> Out2/1

== system Controller_HIL/CAN_Tx/CAN_Data/Selector11 ==
  In1 : Inport
  Bus Creator : BusCreator  Inputs=24
  Demux : Demux  Outputs=100
  Mux1 : Mux  Inputs=76
  Terminator : Terminator
  Out1 : Outport
  wires:
  Demux/1 -> Bus Creator/1
  Demux/2 -> Bus Creator/2
  Demux/3 -> Bus Creator/3
  Demux/4 -> Bus Creator/4
  Demux/5 -> Bus Creator/5
  Demux/6 -> Bus Creator/6
  Demux/7 -> Bus Creator/7
  Demux/8 -> Bus Creator/8
  Demux/9 -> Bus Creator/9
  Demux/10 -> Bus Creator/10
  Demux/11 -> Bus Creator/11
  Demux/12 -> Bus Creator/12
  Demux/13 -> Bus Creator/13
  Demux/14 -> Bus Creator/14
  Demux/15 -> Bus Creator/15
  Demux/16 -> Bus Creator/16
  Demux/17 -> Bus Creator/17
  Demux/18 -> Bus Creator/18
  Demux/19 -> Bus Creator/19
  Demux/20 -> Bus Creator/20
  Demux/21 -> Bus Creator/21
  Demux/22 -> Bus Creator/22
  Demux/23 -> Bus Creator/23
  Demux/24 -> Bus Creator/24
  Demux/25 -> Mux1/1
  Demux/26 -> Mux1/2
  Demux/27 -> Mux1/3
  Demux/28 -> Mux1/4
  Demux/29 -> Mux1/5
  Demux/30 -> Mux1/6
  Demux/31 -> Mux1/7
  Demux/32 -> Mux1/8
  Demux/33 -> Mux1/9
  Demux/34 -> Mux1/10
  Demux/35 -> Mux1/11
  Demux/36 -> Mux1/12
  Demux/37 -> Mux1/13
  Demux/38 -> Mux1/14
  Demux/39 -> Mux1/15
  Demux/40 -> Mux1/16
  Demux/41 -> Mux1/17
  Demux/42 -> Mux1/18
  Demux/43 -> Mux1/19
  Demux/44 -> Mux1/20
  Demux/45 -> Mux1/21
  Demux/46 -> Mux1/22
  Demux/47 -> Mux1/23
  Demux/48 -> Mux1/24
  Demux/49 -> Mux1/25
  Demux/50 -> Mux1/26
  Demux/51 -> Mux1/27
  Demux/52 -> Mux1/28
  Demux/53 -> Mux1/29
  Demux/54 -> Mux1/30
  Demux/55 -> Mux1/31
  Demux/56 -> Mux1/32
  Demux/57 -> Mux1/33
  Demux/58 -> Mux1/34
  Demux/59 -> Mux1/35
  Demux/60 -> Mux1/36
  Demux/61 -> Mux1/37
  Demux/62 -> Mux1/38
  Demux/63 -> Mux1/39
  Demux/64 -> Mux1/40
  Demux/65 -> Mux1/41
  Demux/66 -> Mux1/42
  Demux/67 -> Mux1/43
  Demux/68 -> Mux1/44
  Demux/69 -> Mux1/45
  Demux/70 -> Mux1/46
  Demux/71 -> Mux1/47
  Demux/72 -> Mux1/48
  Demux/73 -> Mux1/49
  Demux/74 -> Mux1/50
  Demux/75 -> Mux1/51
  Demux/76 -> Mux1/52
  Demux/77 -> Mux1/53
  Demux/78 -> Mux1/54
  Demux/79 -> Mux1/55
  Demux/80 -> Mux1/56
  Demux/81 -> Mux1/57
  Demux/82 -> Mux1/58
  Demux/83 -> Mux1/59
  Demux/84 -> Mux1/60
  Demux/85 -> Mux1/61
  Demux/86 -> Mux1/62
  Demux/87 -> Mux1/63
  Demux/88 -> Mux1/64
  Demux/89 -> Mux1/65
  Demux/90 -> Mux1/66
  Demux/91 -> Mux1/67
  Demux/92 -> Mux1/68
  Demux/93 -> Mux1/69
  Demux/94 -> Mux1/70
  Demux/95 -> Mux1/71
  Demux/96 -> Mux1/72
  Demux/97 -> Mux1/73
  Demux/98 -> Mux1/74
  Demux/99 -> Mux1/75
  Demux/100 -> Mux1/76
  Mux1/1 -> Out1/1
  Bus Creator/1 -> Terminator/1
  In1/1 -> Demux/1

== system Controller_HIL/Controller/Controller/BMS State Machine ==
  Discharge_Current_Limit : Inport
  Charge_Current_Limit : Inport  Port=2
  State_Request : Inport  Port=3  OutDataTypeStr=Enum: SRE
  Sensor_Values : Inport  Port=4
  Fault_Reset_Enable : Inport  Port=5
  Bus Selector : BusSelector  OutputSignals=Cell_Voltages,Pack_Voltage,Cell_Temperatures,Pack_Current
  Data Type Conversion : DataTypeConversion  OutDataTypeStr=boolean  SaturateOnIntegerOverflow=off  RndMeth=Floor
  State_Machine : Stateflow chart  TreatAsAtomicUnit=on  VariantControl=(default)
  Charge_Current_Req : Outport  OutMin=-100  OutMax=100  OutDataTypeStr=single  VectorParamsAs1DForOutWhenUnconnected=off
  Faults : Outport  Port=2  OutDataTypeStr=Bus: Faults  VectorParamsAs1DForOutWhenUnconnected=off  BusOutputAsStruct=on
  Charging_State : Outport  Port=3
  BMS_State : Outport  Port=4  OutDataTypeStr=Enum: BMS_Controller_State  VectorParamsAs1DForOutWhenUnconnected=off
  wires:
  State_Machine/2(Fault_out) -> Faults/1  "Faults"
  Bus Selector/1 -> State_Machine/4(Cell_Voltages)  "<Cell_Voltages>"
  State_Machine/1(ChargeCurrentReq) -> Charge_Current_Req/1  "Charge_Current_Req"
  State_Request/1 -> State_Machine/3(State_Request)
  Discharge_Current_Limit/1 -> State_Machine/1(DischargeCurrentLimit)
  Charge_Current_Limit/1 -> State_Machine/2(ChargeCurrentLimit)
  Bus Selector/3 -> State_Machine/6(Cell_Temperatures)  "<Cell_Temperatures>"
  Bus Selector/2 -> State_Machine/5(Pack_Voltage)  "<Pack_Voltage>"
  Bus Selector/4 -> State_Machine/7(Pack_Current)  "<Pack_Current>"
  Sensor_Values/1 -> Bus Selector/1
  Fault_Reset_Enable/1 -> Data Type Conversion/1
  Data Type Conversion/1 -> State_Machine/8(Fault_Reset_Enable)
  State_Machine/3(ChargeModeReq) -> Charging_State/1  "Charging_State"
  State_Machine/4(BMS_State) -> BMS_State/1  "BMS_State"

== system Controller_HIL/Controller/Controller/Balancing Logic ==
  BMS_State : Inport  OutDataTypeStr=Enum: BMS_Controller_State  PortDimensions=1
  Sensor_Values : Inport  Port=2
  Balancing : Stateflow chart  TreatAsAtomicUnit=on  VariantControl=(default)
  Bus Selector1 : BusSelector  OutputSignals=Cell_Voltages
  Bal_Cmd : Outport  OutDataTypeStr=boolean  PortDimensions=[1,NumModules*Ns_Module]  VectorParamsAs1DForOutWhenUnconnected=off
  wires:
  Balancing/1(Bal_Cmd) -> Bal_Cmd/1  "Bal_Cmd"
  Bus Selector1/1 -> Balancing/2(CellVoltages)  "<Cell_Voltages>"
  Sensor_Values/1 -> Bus Selector1/1
  BMS_State/1 -> Balancing/1(BMS_State)

== system Controller_HIL/Controller/Controller/Current Calculations ==
  BMS_Input : Inport
  Bus Selector : BusSelector  OutputSignals=Cell_Voltages,Cell_Temperatures
  Charge_Current_Limit_Calc : Subsystem
  Discharge_Current_Limit_Calc : Subsystem
  MinMax : MinMax
  MinMax1 : MinMax
  MinMax2 : MinMax  Function=max
  MinMax4 : MinMax  Function=max
  Discharge_Current_Limit : Outport
  Charge_Current_Limit : Outport  Port=2
  wires:
  MinMax/1 -> Discharge_Current_Limit_Calc/1(MinCellVolt)  "Min_Cell_Volt"
  MinMax4/1 -> Discharge_Current_Limit_Calc/3(MaxCellTemp), Charge_Current_Limit_Calc/3(MaxCellTemp)  "Max_Cell_Temp"
  MinMax1/1 -> Discharge_Current_Limit_Calc/2(MinCellTemp), Charge_Current_Limit_Calc/2(MinCellTemp)  "Min_Cell_Temp"
  MinMax2/1 -> Charge_Current_Limit_Calc/1(MaxCellVolt)  "Max_Cell_Volt"
  Discharge_Current_Limit_Calc/1(Discharge_Current_Limit) -> Discharge_Current_Limit/1  "Discharge_Current_Limit"
  Charge_Current_Limit_Calc/1(Charge_Current_Limit) -> Charge_Current_Limit/1  "Charge_Current_Limit"
  Bus Selector/1 -> MinMax/1, MinMax2/1  "<Cell_Voltages>"
  Bus Selector/2 -> MinMax4/1, MinMax1/1  "<Cell_Temperatures>"
  BMS_Input/1 -> Bus Selector/1

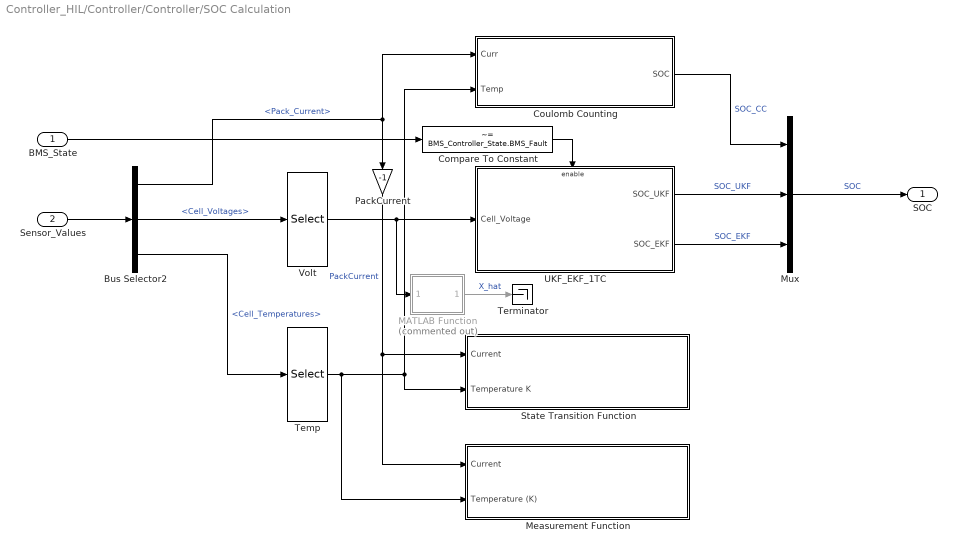
== system Controller_HIL/Controller/Controller/SOC Calculation ==
  BMS_State : Inport  OutDataTypeStr=Enum: BMS_Controller_State
  Sensor_Values : Inport  Port=2
  Bus Selector2 : BusSelector  OutputSignals=Pack_Current,Cell_Voltages,Cell_Temperatures
  Compare To Constant : simulink/Logic and Bit Operations/Compare To Constant  relop=~=  const=BMS_Controller_State.BMS_Fault  OutDataTypeStr=boolean
  Coulomb Counting : Subsystem  VariantControl=SocAlgo==1
  MATLAB Function : MATLAB Function  Commented=on  TreatAsAtomicUnit=on
  Measurement Function : Subsystem  TreatAsAtomicUnit=on
  Mux : Mux  Inputs=3
  PackCurrent : Gain  Gain=-1
  State Transition Function : Subsystem  TreatAsAtomicUnit=on
  Temp : Selector  InputPortWidth=Ns_Module*NumModules  IndexOptions=Index vector (dialog)  Indices=1  OutputSizes=1
  Terminator : Terminator
  UKF_EKF_1TC : Subsystem  VariantControl=CellType==1
  Volt : Selector  InputPortWidth=Ns_Module*NumModules  IndexOptions=Index vector (dialog)  Indices=1  OutputSizes=1
  SOC : Outport  OutDataTypeStr=single  VectorParamsAs1DForOutWhenUnconnected=off
  wires:
  Mux/1 -> SOC/1  "SOC"
  UKF_EKF_1TC/1(SOC_UKF) -> Mux/2  "SOC_UKF"
  BMS_State/1 -> Compare To Constant/1
  Coulomb Counting/1(SOC) -> Mux/1  "SOC_CC"
  Volt/1 -> MATLAB Function/1(meas), UKF_EKF_1TC/1(Cell_Voltage)
  MATLAB Function/1(xhatOut) -> Terminator/1  "X_hat"
  Temp/1 -> Coulomb Counting/2(Temp), State Transition Function/2(Temperature K), Measurement Function/2(Temperature (K))
  Compare To Constant/1 -> UKF_EKF_1TC/Enable
  UKF_EKF_1TC/2(SOC_EKF) -> Mux/3  "SOC_EKF"
  Bus Selector2/1 -> Coulomb Counting/1(Curr), PackCurrent/1  "<Pack_Current>"
  PackCurrent/1 -> State Transition Function/1(Current), Measurement Function/1(Current)  "PackCurrent"
  Bus Selector2/3 -> Temp/1  "<Cell_Temperatures>"
  Bus Selector2/2 -> Volt/1  "<Cell_Voltages>"
  Sensor_Values/1 -> Bus Selector2/1

== system Controller_HIL/CAN Rx/RX_FIFO_Complete_Event/Temperature/Action_Rx_0x1 ==
  Data : Inport
  Action Port : ActionPort  ActionPortLabel=case [ 1032 ]:
  Byte Unpack : etargetslib/Byte Unpack  dimensions={[1] [1]}  datatypes={'single', 'single'}  byteAlign=1
      settings: LibrarySourceBlock=embeddedtargetslib/Host Communication/Byte Unpack
  FCAN_Receive_FIFO : mbd_s32k1xx_ec_toolbox/Communication Blocks/CAN Blocks/FCAN_Receive  can_instance=0  can_mode=Non-blocking  can_timeout_ms=0  can_mb_idx=0  can_mb_init=Once  show_id_input=off  can_extended_id=off  can_is_remote=off  can_id=0x7FF  can_msg_mask=0  show_adv_opts=on  can_use_rxfifo=on  can_fd_enable=off
  Outport : Outport
  Outport1 : Outport  Port=2
  wires:
  Data/1 -> Byte Unpack/1
  Byte Unpack/1 -> Outport/1
  Byte Unpack/2 -> Outport1/1

== system Controller_HIL/CAN Rx/RX_FIFO_Complete_Event/Temperature/Action_Rx_0x10 ==
  Data : Inport
  Action Port : ActionPort  ActionPortLabel=case [ 1047 ]:
  Byte Unpack : etargetslib/Byte Unpack  dimensions={[1] [1]}  datatypes={'single', 'single'}  byteAlign=1
      settings: LibrarySourceBlock=embeddedtargetslib/Host Communication/Byte Unpack
  FCAN_Receive_FIFO : mbd_s32k1xx_ec_toolbox/Communication Blocks/CAN Blocks/FCAN_Receive  can_instance=0  can_mode=Non-blocking  can_timeout_ms=0  can_mb_idx=0  can_mb_init=Once  show_id_input=off  can_extended_id=off  can_is_remote=off  can_id=0x7FF  can_msg_mask=0  show_adv_opts=on  can_use_rxfifo=on  can_fd_enable=off
  Outport : Outport
  Outport1 : Outport  Port=2
  wires:
  Data/1 -> Byte Unpack/1
  Byte Unpack/1 -> Outport/1
  Byte Unpack/2 -> Outport1/1

== system Controller_HIL/CAN Rx/RX_FIFO_Complete_Event/Temperature/Action_Rx_0x11 ==
  Data : Inport
  Action Port : ActionPort  ActionPortLabel=case [ 1048 ]:
  Byte Unpack : etargetslib/Byte Unpack  dimensions={[1] [1]}  datatypes={'single', 'single'}  byteAlign=1
      settings: LibrarySourceBlock=embeddedtargetslib/Host Communication/Byte Unpack
  FCAN_Receive_FIFO : mbd_s32k1xx_ec_toolbox/Communication Blocks/CAN Blocks/FCAN_Receive  can_instance=0  can_mode=Non-blocking  can_timeout_ms=0  can_mb_idx=0  can_mb_init=Once  show_id_input=off  can_extended_id=off  can_is_remote=off  can_id=0x7FF  can_msg_mask=0  show_adv_opts=on  can_use_rxfifo=on  can_fd_enable=off
  Outport : Outport
  Outport1 : Outport  Port=2
  wires:
  Data/1 -> Byte Unpack/1
  Byte Unpack/2 -> Outport1/1
  Byte Unpack/1 -> Outport/1

== system Controller_HIL/CAN Rx/RX_FIFO_Complete_Event/Temperature/Action_Rx_0x12 ==
  Data : Inport
  Action Port : ActionPort  ActionPortLabel=case [ 1049 ]:
  Byte Unpack : etargetslib/Byte Unpack  dimensions={[1] [1]}  datatypes={'single', 'single'}  byteAlign=1
      settings: LibrarySourceBlock=embeddedtargetslib/Host Communication/Byte Unpack
  FCAN_Receive_FIFO : mbd_s32k1xx_ec_toolbox/Communication Blocks/CAN Blocks/FCAN_Receive  can_instance=0  can_mode=Non-blocking  can_timeout_ms=0  can_mb_idx=0  can_mb_init=Once  show_id_input=off  can_extended_id=off  can_is_remote=off  can_id=0x7FF  can_msg_mask=0  show_adv_opts=on  can_use_rxfifo=on  can_fd_enable=off
  Outport : Outport
  Outport1 : Outport  Port=2
  wires:
  Byte Unpack/1 -> Outport/1
  Byte Unpack/2 -> Outport1/1
  Data/1 -> Byte Unpack/1

== system Controller_HIL/CAN Rx/RX_FIFO_Complete_Event/Temperature/Action_Rx_0x13 ==
  Data : Inport
  Action Port : ActionPort  ActionPortLabel=case [ 1056 ]:
  Byte Unpack : etargetslib/Byte Unpack  dimensions={[1] [1]}  datatypes={'single', 'single'}  byteAlign=1
      settings: LibrarySourceBlock=embeddedtargetslib/Host Communication/Byte Unpack
  FCAN_Receive_FIFO : mbd_s32k1xx_ec_toolbox/Communication Blocks/CAN Blocks/FCAN_Receive  can_instance=0  can_mode=Non-blocking  can_timeout_ms=0  can_mb_idx=0  can_mb_init=Once  show_id_input=off  can_extended_id=off  can_is_remote=off  can_id=0x7FF  can_msg_mask=0  show_adv_opts=on  can_use_rxfifo=on  can_fd_enable=off
  Outport : Outport
  Outport1 : Outport  Port=2
  wires:
  Data/1 -> Byte Unpack/1
  Byte Unpack/1 -> Outport/1
  Byte Unpack/2 -> Outport1/1

== system Controller_HIL/CAN Rx/RX_FIFO_Complete_Event/Temperature/Action_Rx_0x14 ==
  Data : Inport
  Action Port : ActionPort  ActionPortLabel=case [ 1057 ]:
  Byte Unpack : etargetslib/Byte Unpack  dimensions={[1] [1]}  datatypes={'single', 'single'}  byteAlign=1
      settings: LibrarySourceBlock=embeddedtargetslib/Host Communication/Byte Unpack
  FCAN_Receive_FIFO : mbd_s32k1xx_ec_toolbox/Communication Blocks/CAN Blocks/FCAN_Receive  can_instance=0  can_mode=Non-blocking  can_timeout_ms=0  can_mb_idx=0  can_mb_init=Once  show_id_input=off  can_extended_id=off  can_is_remote=off  can_id=0x7FF  can_msg_mask=0  show_adv_opts=on  can_use_rxfifo=on  can_fd_enable=off
  Outport : Outport
  Outport1 : Outport  Port=2
  wires:
  Data/1 -> Byte Unpack/1
  Byte Unpack/2 -> Outport1/1
  Byte Unpack/1 -> Outport/1

== system Controller_HIL/CAN Rx/RX_FIFO_Complete_Event/Temperature/Action_Rx_0x15 ==
  Data : Inport
  Action Port : ActionPort  ActionPortLabel=case [ 1058 ]:
  Byte Unpack : etargetslib/Byte Unpack  dimensions={[1] [1]}  datatypes={'single', 'single'}  byteAlign=1
      settings: LibrarySourceBlock=embeddedtargetslib/Host Communication/Byte Unpack
  FCAN_Receive_FIFO : mbd_s32k1xx_ec_toolbox/Communication Blocks/CAN Blocks/FCAN_Receive  can_instance=0  can_mode=Non-blocking  can_timeout_ms=0  can_mb_idx=0  can_mb_init=Once  show_id_input=off  can_extended_id=off  can_is_remote=off  can_id=0x7FF  can_msg_mask=0  show_adv_opts=on  can_use_rxfifo=on  can_fd_enable=off
  Outport : Outport
  Outport1 : Outport  Port=2
  wires:
  Byte Unpack/1 -> Outport/1
  Byte Unpack/2 -> Outport1/1
  Data/1 -> Byte Unpack/1

== system Controller_HIL/CAN Rx/RX_FIFO_Complete_Event/Temperature/Action_Rx_0x16 ==
  Data : Inport
  Action Port : ActionPort  ActionPortLabel=case [ 1059 ]:
  Byte Unpack : etargetslib/Byte Unpack  dimensions={[1] [1]}  datatypes={'single', 'single'}  byteAlign=1
      settings: LibrarySourceBlock=embeddedtargetslib/Host Communication/Byte Unpack
  FCAN_Receive_FIFO : mbd_s32k1xx_ec_toolbox/Communication Blocks/CAN Blocks/FCAN_Receive  can_instance=0  can_mode=Non-blocking  can_timeout_ms=0  can_mb_idx=0  can_mb_init=Once  show_id_input=off  can_extended_id=off  can_is_remote=off  can_id=0x7FF  can_msg_mask=0  show_adv_opts=on  can_use_rxfifo=on  can_fd_enable=off
  Outport : Outport
  Outport1 : Outport  Port=2
  wires:
  Data/1 -> Byte Unpack/1
  Byte Unpack/1 -> Outport/1
  Byte Unpack/2 -> Outport1/1

== system Controller_HIL/CAN Rx/RX_FIFO_Complete_Event/Temperature/Action_Rx_0x17 ==
  Data : Inport
  Action Port : ActionPort  ActionPortLabel=case [ 1060 ]:
  Byte Unpack : etargetslib/Byte Unpack  dimensions={[1] [1]}  datatypes={'single', 'single'}  byteAlign=1
      settings: LibrarySourceBlock=embeddedtargetslib/Host Communication/Byte Unpack
  FCAN_Receive_FIFO : mbd_s32k1xx_ec_toolbox/Communication Blocks/CAN Blocks/FCAN_Receive  can_instance=0  can_mode=Non-blocking  can_timeout_ms=0  can_mb_idx=0  can_mb_init=Once  show_id_input=off  can_extended_id=off  can_is_remote=off  can_id=0x7FF  can_msg_mask=0  show_adv_opts=on  can_use_rxfifo=on  can_fd_enable=off
  Outport : Outport
  Outport1 : Outport  Port=2
  wires:
  Data/1 -> Byte Unpack/1
  Byte Unpack/2 -> Outport1/1
  Byte Unpack/1 -> Outport/1

== system Controller_HIL/CAN Rx/RX_FIFO_Complete_Event/Temperature/Action_Rx_0x18 ==
  Data : Inport
  Action Port : ActionPort  ActionPortLabel=case [ 1061 ]:
  Byte Unpack : etargetslib/Byte Unpack  dimensions={[1] [1]}  datatypes={'single', 'single'}  byteAlign=1
      settings: LibrarySourceBlock=embeddedtargetslib/Host Communication/Byte Unpack
  FCAN_Receive_FIFO : mbd_s32k1xx_ec_toolbox/Communication Blocks/CAN Blocks/FCAN_Receive  can_instance=0  can_mode=Non-blocking  can_timeout_ms=0  can_mb_idx=0  can_mb_init=Once  show_id_input=off  can_extended_id=off  can_is_remote=off  can_id=0x7FF  can_msg_mask=0  show_adv_opts=on  can_use_rxfifo=on  can_fd_enable=off
  Outport : Outport
  Outport1 : Outport  Port=2
  wires:
  Byte Unpack/1 -> Outport/1
  Byte Unpack/2 -> Outport1/1
  Data/1 -> Byte Unpack/1

== system Controller_HIL/CAN Rx/RX_FIFO_Complete_Event/Temperature/Action_Rx_0x19 ==
  Data : Inport
  Action Port : ActionPort  ActionPortLabel=case [ 1062 ]:
  Byte Unpack : etargetslib/Byte Unpack  dimensions={[1] [1]}  datatypes={'single', 'single'}  byteAlign=1
      settings: LibrarySourceBlock=embeddedtargetslib/Host Communication/Byte Unpack
  FCAN_Receive_FIFO : mbd_s32k1xx_ec_toolbox/Communication Blocks/CAN Blocks/FCAN_Receive  can_instance=0  can_mode=Non-blocking  can_timeout_ms=0  can_mb_idx=0  can_mb_init=Once  show_id_input=off  can_extended_id=off  can_is_remote=off  can_id=0x7FF  can_msg_mask=0  show_adv_opts=on  can_use_rxfifo=on  can_fd_enable=off
  Outport : Outport
  Outport1 : Outport  Port=2
  wires:
  Data/1 -> Byte Unpack/1
  Byte Unpack/1 -> Outport/1
  Byte Unpack/2 -> Outport1/1
